simulink model "MartLowTempMechanicalModel"  (R2018a)
settings: Solver=FixedStepAuto  StartTime=0.0  StopTime=10.0  FixedStep=10e-6  RelTol=1e-3
values from neighbouring files (symbols this model uses):
  temp = temp_range(i)    [MartLowTempRunner.m]
undefined symbols (not defined in the file or in its folder): cSf, cSs, Da, Dm, rEmax, Theta
settings Model: Creator=Michau  LastModifiedBy=Michau
settings SolverCC: AlgebraicLoopSolver=LineSearch

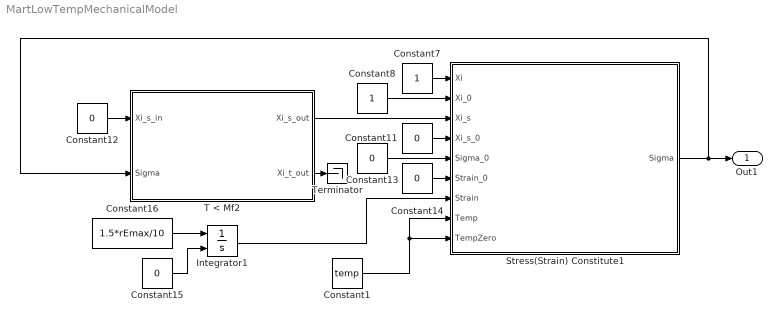
== system MartLowTempMechanicalModel ==
  Constant1 : Constant  Value=temp
  Constant{11..15} (5 alike) : Constant  Value=0
  Constant16 : Constant  Value=1.5*rEmax/10
  Constant7 : Constant
  Constant8 : Constant
  Integrator1 : Integrator  InitialConditionSource=external
  Stress(Strain) Constitute1 : Subsystem
  T < Mf2 : Subsystem
  Terminator : Terminator
  Out1 : Outport
  wires:
  Constant16/1 -> Integrator1/1
  Integrator1/1 -> Stress(Strain) Constitute1/7(Strain)
  T < Mf2/1(Xi_s_out) -> Stress(Strain) Constitute1/3(Xi_s)
  Constant12/1 -> T < Mf2/1(Xi_s_in)
  Stress(Strain) Constitute1/1(Sigma) -> Out1/1, T < Mf2/2(Sigma)
  Constant15/1 -> Integrator1/2
  Constant14/1 -> Stress(Strain) Constitute1/6(Strain_0)
  Constant13/1 -> Stress(Strain) Constitute1/5(Sigma_0)
  Constant7/1 -> Stress(Strain) Constitute1/1(Xi)
  Constant11/1 -> Stress(Strain) Constitute1/4(Xi_s_0)
  Constant8/1 -> Stress(Strain) Constitute1/2(Xi_0)
  Constant1/1 -> Stress(Strain) Constitute1/9(TempZero), Stress(Strain) Constitute1/8(Temp)
  T < Mf2/2("Xi_t_out ") -> Terminator/1

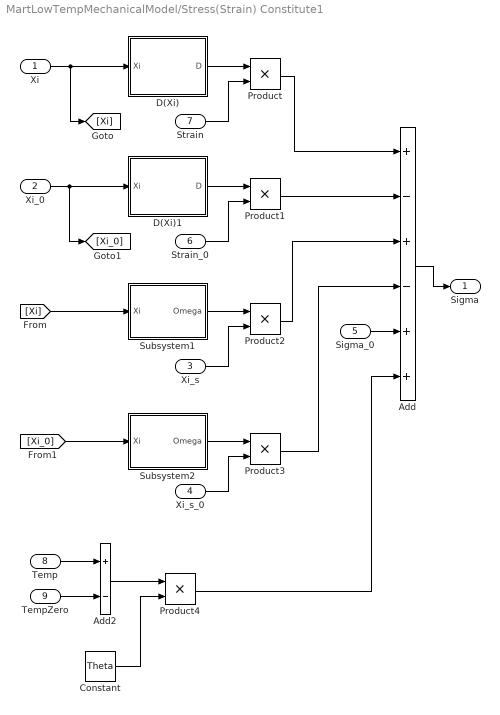
== system MartLowTempMechanicalModel/Stress(Strain) Constitute1 ==
  Xi : Inport
  Xi_0 : Inport  Port=2
  Xi_s : Inport  Port=3
  Xi_s_0 : Inport  Port=4
  Sigma_0 : Inport  Port=5
  Strain_0 : Inport  Port=6
  Strain : Inport  Port=7
  Temp : Inport  Port=8
  TempZero : Inport  Port=9
  Add : Sum  Inputs=+-+-++
  Add2 : Sum  Inputs=+-
  Constant : Constant  Value=Theta
  D(Xi) : Subsystem
  D(Xi)1 : Subsystem
  Product{,1..4} (5 alike) : Product
  Subsystem1 : Subsystem
  Subsystem2 : Subsystem
  Sigma : Outport
  wires:
  Xi/1 -> [Xi], D(Xi)/1(Xi)
  D(Xi)/1(D) -> Product/1
  Strain/1 -> Product/2
  Xi_0/1 -> [Xi_0], D(Xi)1/1(Xi)
  D(Xi)1/1(D) -> Product1/1
  Strain_0/1 -> Product1/2
  [Xi] -> Subsystem1/1(Xi)
  Subsystem1/1(Omega) -> Product2/1
  Xi_s/1 -> Product2/2
  [Xi_0] -> Subsystem2/1(Xi)
  Subsystem2/1(Omega) -> Product3/1
  Xi_s_0/1 -> Product3/2
  Product/1 -> Add/1
  Product1/1 -> Add/2
  Product2/1 -> Add/3
  Product3/1 -> Add/4
  Sigma_0/1 -> Add/5
  Add/1 -> Sigma/1
  TempZero/1 -> Add2/2
  Temp/1 -> Add2/1
  Product4/1 -> Add/6
  Add2/1 -> Product4/1
  Constant/1 -> Product4/2

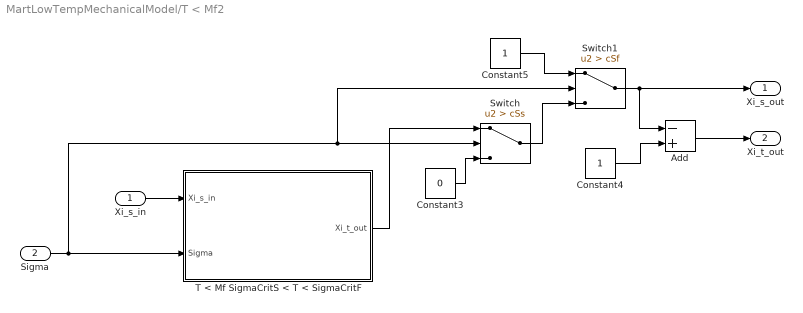
== system MartLowTempMechanicalModel/T < Mf2 ==
  Xi_s_in : Inport
  Sigma : Inport  Port=2
  Add : Sum  Inputs=-+
  Constant3 : Constant  Value=0
  Constant4 : Constant
  Constant5 : Constant
  Switch : Switch  Criteria=u2 > Threshold  Threshold=cSs
  Switch1 : Switch  Criteria=u2 > Threshold  Threshold=cSf
  T < Mf SigmaCritS < T < SigmaCritF : Subsystem
  Xi_s_out : Outport
  "Xi_t_out " : Outport  Port=2
  wires:
  Constant3/1 -> Switch/3
  Sigma/1 -> Switch/2, Switch1/2, T < Mf SigmaCritS < T < SigmaCritF/2(Sigma)
  Switch/1 -> Switch1/3
  T < Mf SigmaCritS < T < SigmaCritF/1(Xi_t_out) -> Switch/1
  Xi_s_in/1 -> T < Mf SigmaCritS < T < SigmaCritF/1(Xi_s_in)
  Constant4/1 -> Add/2
  Switch1/1 -> Xi_s_out/1, Add/1
  Constant5/1 -> Switch1/1
  Add/1 -> "Xi_t_out "/1

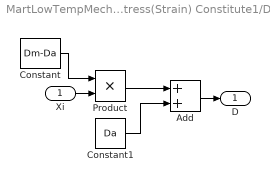
== system MartLowTempMechanicalModel/Stress(Strain) Constitute1/D(Xi) ==
  Xi : Inport
  Add : Sum
  Constant : Constant  Value=Dm-Da
  Constant1 : Constant  Value=Da
  Product : Product
  D : Outport
  wires:
  Xi/1 -> Product/2
  Product/1 -> Add/1
  Constant1/1 -> Add/2
  Constant/1 -> Product/1
  Add/1 -> D/1

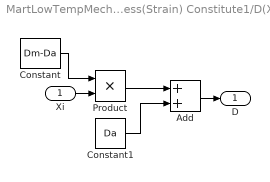
== system MartLowTempMechanicalModel/Stress(Strain) Constitute1/D(Xi)1 ==
  Xi : Inport
  Add : Sum
  Constant : Constant  Value=Dm-Da
  Constant1 : Constant  Value=Da
  Product : Product
  D : Outport
  wires:
  Xi/1 -> Product/2
  Product/1 -> Add/1
  Constant1/1 -> Add/2
  Constant/1 -> Product/1
  Add/1 -> D/1

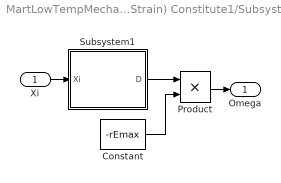
== system MartLowTempMechanicalModel/Stress(Strain) Constitute1/Subsystem1 ==
  Xi : Inport
  Constant : Constant  Value=-rEmax
  Product : Product
  Subsystem1 : Subsystem
  Omega : Outport
  wires:
  Product/1 -> Omega/1
  Subsystem1/1(D) -> Product/1
  Constant/1 -> Product/2
  Xi/1 -> Subsystem1/1(Xi)

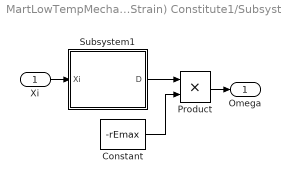
== system MartLowTempMechanicalModel/Stress(Strain) Constitute1/Subsystem2 ==
  Xi : Inport
  Constant : Constant  Value=-rEmax
  Product : Product
  Subsystem1 : Subsystem
  Omega : Outport
  wires:
  Product/1 -> Omega/1
  Subsystem1/1(D) -> Product/1
  Constant/1 -> Product/2
  Xi/1 -> Subsystem1/1(Xi)

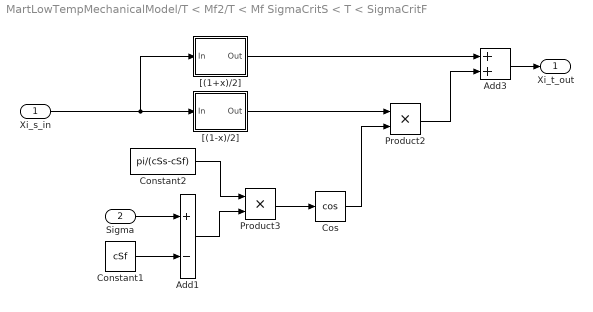
== system MartLowTempMechanicalModel/T < Mf2/T < Mf SigmaCritS < T < SigmaCritF ==
  Xi_s_in : Inport
  Sigma : Inport  Port=2
  Add1 : Sum  Inputs=+-
  Add3 : Sum
  Constant1 : Constant  Value=cSf
  Constant2 : Constant  Value=pi/(cSs-cSf)
  Cos : Trigonometry  Operator=cos
  Product2 : Product
  Product3 : Product
  "[(1+x)/2]" : Subsystem
  "[(1-x)/2]" : Subsystem
  Xi_t_out : Outport
  wires:
  Cos/1 -> Product2/2
  Product2/1 -> Add3/2
  Add1/1 -> Product3/2
  Sigma/1 -> Add1/1
  Add3/1 -> Xi_t_out/1
  Xi_s_in/1 -> "[(1+x)/2]"/1(In), "[(1-x)/2]"/1(In)
  Product3/1 -> Cos/1
  "[(1+x)/2]"/1(Out) -> Add3/1
  "[(1-x)/2]"/1(Out) -> Product2/1
  Constant2/1 -> Product3/1
  Constant1/1 -> Add1/2

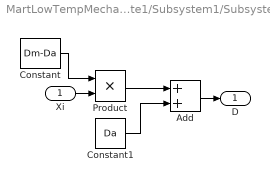
== system MartLowTempMechanicalModel/Stress(Strain) Constitute1/Subsystem1/Subsystem1 ==
  Xi : Inport
  Add : Sum
  Constant : Constant  Value=Dm-Da
  Constant1 : Constant  Value=Da
  Product : Product
  D : Outport
  wires:
  Xi/1 -> Product/2
  Product/1 -> Add/1
  Constant1/1 -> Add/2
  Constant/1 -> Product/1
  Add/1 -> D/1

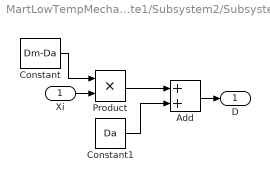
== system MartLowTempMechanicalModel/Stress(Strain) Constitute1/Subsystem2/Subsystem1 ==
  Xi : Inport
  Add : Sum
  Constant : Constant  Value=Dm-Da
  Constant1 : Constant  Value=Da
  Product : Product
  D : Outport
  wires:
  Xi/1 -> Product/2
  Product/1 -> Add/1
  Constant1/1 -> Add/2
  Constant/1 -> Product/1
  Add/1 -> D/1

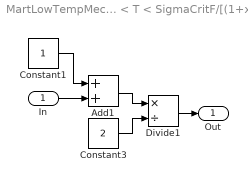
== system MartLowTempMechanicalModel/T < Mf2/T < Mf SigmaCritS < T < SigmaCritF/[(1+x)//2] ==
  In : Inport
  Add1 : Sum
  Constant1 : Constant
  Constant3 : Constant  Value=2
  Divide1 : Product  Inputs=*/
  Out : Outport
  wires:
  Constant3/1 -> Divide1/2
  Divide1/1 -> Out/1
  Constant1/1 -> Add1/1
  In/1 -> Add1/2
  Add1/1 -> Divide1/1

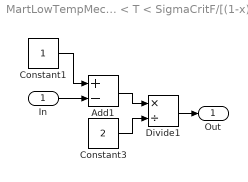
== system MartLowTempMechanicalModel/T < Mf2/T < Mf SigmaCritS < T < SigmaCritF/[(1-x)//2] ==
  In : Inport
  Add1 : Sum  Inputs=+-
  Constant1 : Constant
  Constant3 : Constant  Value=2
  Divide1 : Product  Inputs=*/
  Out : Outport
  wires:
  Constant3/1 -> Divide1/2
  Divide1/1 -> Out/1
  Constant1/1 -> Add1/1
  In/1 -> Add1/2
  Add1/1 -> Divide1/1
